simulink model "ManualModel_With_OptiTrack"  (R2025a)
settings: Solver=ode4  StartTime=0  StopTime=inf  FixedStep=0.01  RelTol=1e-3
undefined symbols (not defined in the file): Angular, getRigidBodyPose, Linear, scenario
libraries: robotlib x4, simulink_extras x2, vrlib x1
settings Model: SimulationMode=external  Creator=20212285  LastModifiedBy=jakub
settings SolverCC: AlgebraicLoopSolver=LineSearch
settings DataIOCC: ReturnWorkspaceOutputsName=s
settings OptimizationCC: EnhancedBackFolding=on  PassReuseOutputArgsAs=Individual arguments  ZeroExternalMemoryAtStartup=off  ZeroInternalMemoryAtStartup=off  MaxStackSize=64  OptimizeBlockOrder=speed  DifferentSizesBufferReuse=on  OptimizationCustomize=off  EfficientTunableParamExpr=on
settings DebuggingCC: ParameterTunabilityLossMsg=error  UnconnectedInputMsg=warning  UnconnectedOutputMsg=warning  UnconnectedLineMsg=warning
settings HardwareCC: ProdBitPerPointer=32.0  ProdBitPerSizeT=32.0  ProdBitPerPtrDiffT=32.0  ProdLargestAtomicFloat=None  ProdIntDivRoundTo=Undefined  ProdEndianess=Unspecified  ProdWordSize=32.0  ProdHWDeviceType=Generic->Unspecified (assume 32-bit Generic)
settings ModelReferenceCC: EnableRefExpFcnMdlSchedulingChecks=on
settings SFSimCC: MATLABDynamicMemAlloc=off  SimTargetLang=C++  SimDLTargetLibrary=mkl-dnn
settings RTWCC: SystemTargetFile=ert.tlc  HardwareBoard=Robot Operating System (ROS)  TLCOptions="-aInlineSetEventsForThisBaseRateFcn=TLC_FALSE -aSuppressMultiTaskScheduler=TLC_FALSE  -aRateBasedStepFcn=0"  TemplateMakefile=ert_default_tmf  Toolchain=Catkin  TargetLang=C++  GPUComputeCapability=3.5  Description=Embedded Coder
settings CodeAppCC: ForceParamTrailComments=on  IgnoreCustomStorageClasses=off  OperatorAnnotations=on  SimulinkDataObjDesc=on  SFDataObjDesc=on  InsertBlockDesc=on
settings ERTTargetCC: ExtModeTransport=0.0  ExtModeStaticAlloc=off  ExtModeMexFile=ext_comm  ExtModeIntrfLevel=Level1  InlinedParameterPlacement=Hierarchical  DynamicArrayContainerType=coder::array

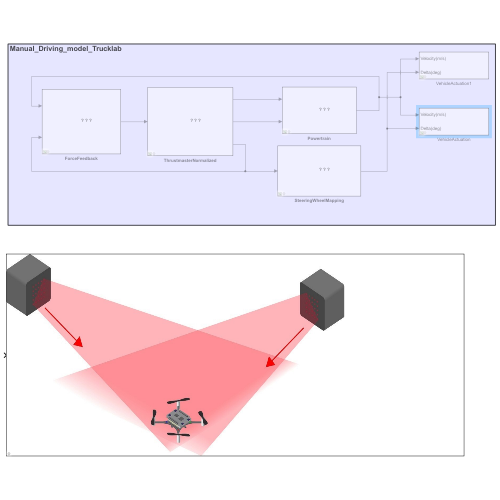
[thumbnail: Simulink's stored preview of the top-level diagram]
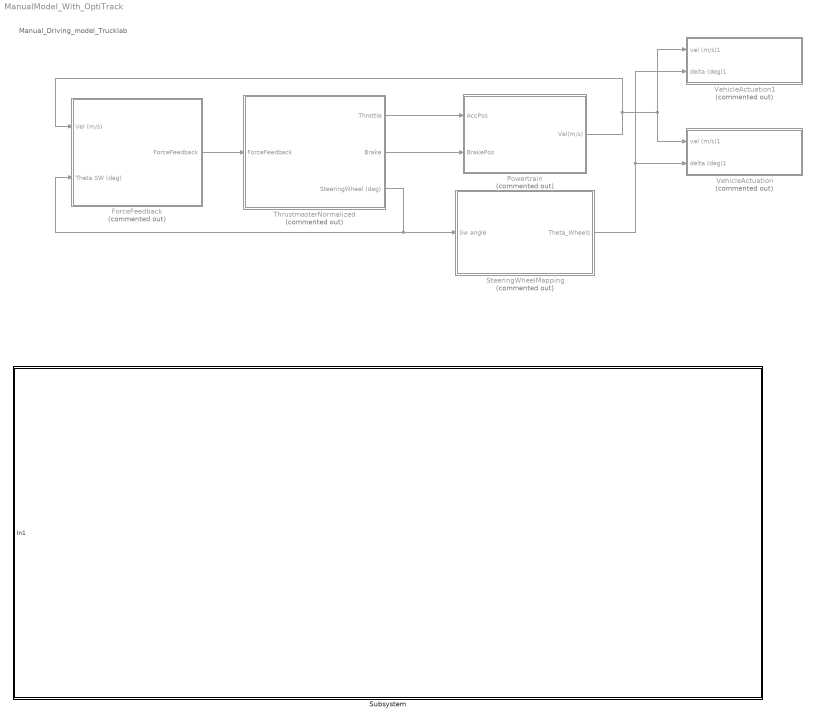
== system ManualModel_With_OptiTrack ==
  note: Manual_Driving_model_Trucklab
  ForceFeedback : Subsystem  Commented=on  mask(Thrustmaster ForceFeedback){}
      mask help:
      | Use this block to give drivers a realistic, centered steer feel: no force at zero.
      |
      | The ForceFeedback block computes a normalized return-to-center torque for a steering wheel. A zero output produces no force; negative values apply maximum rightward torque (–1), and positive values apply maximum leftward torque (+1). Internally, it:
      |
      | Ignores small angles around center (dead-zone)
      | Adds a speed-scaled spring torque pulling the wheel back toward center
      mask Display:
      | image('ForceFeedback.jpg');
      | port_label('input', 1, 'Vel (m/s)')
      | port_label('input', 2, 'Theta_SW (deg)')
      | port_label('output', 1, 'ForceFeedback')
  Powertrain : Subsystem  Commented=on  mask(Powertrain){}
      mask help:
      | Converts driver inputs (Throttle and Brake) and current vehicle speed into longitudinal acceleration. The block outputs a computed acceleration value, which feeds an integrator to produce vehicle velocity, and also outputs a stop_signal that can be used to force the vehicle to halt under very low velocity.
      |
      | Input throttle and brake should be normalized [0,1].
      mask Display:
      | image('Powertrain.jpg');
      | port_label('input', 1, 'Throttle')
      | port_label('input', 2, 'Brake')
      | port_label('output', 1, 'vel (m/s)')
  SteeringWheelMapping : Subsystem  Commented=on  mask(SteeringWheel_Mapping){}
      mask help:
      | SteeringWheel_Mapping maps the raw steering wheel angle (theta_sw) to a modified output (theta_mapped) using one of two modes:
      |
      | Mode = 0 applies a fixed linear gain of 38
      | Mode = 1 applies a nonlinear mapping via the VariableMap function.
      |
      | To change the modes, click the arrow in the bottemleft to open the system, and double-click the manual switch.
      mask Display:
      | image('Steering_mapping.jpg');
      | port_label('input', 1, 'SW_angle (deg)')
      | port_label('output', 1, 'Theta_Wheels (deg)')
  Subsystem : Subsystem
      mask Display: image('optitrack.jpg');
  ThrustmasterNormalized : Subsystem  Commented=on  mask(Thrustmaster_Normalized_Input){}
      mask help:
      | The Thrustmaster_Normalized block converts raw joystick signals from a Thrustmaster wheel‐pedal set into three normalized outputs and one normalized input for force feedback.
      |
      | SteeringWheel output ranges from –450 (full right) to +450 (full left), using standard ISO coordinates (counterclockwise rotation is positive).
      |
      | Pedal (Throttle) output ranges from 0 (no throttle) to 1 (full throttle) using the rightmost pedal.
      |
      | Brake output ranges from 0 (no braking) to 1 (full braking) using the middle pedal.
      |
      | ForceFeedback input accepts a command in the range –1 to +1 to drive the wheel motor.
      mask Display:
      | %image('C:\Users\tarun\OneDrive\Desktop\Flags\thrust.jpg'); % Use "Edit Image" on toolstrip to change.
      | image('joystick.jpg');
      | port_label('input', 1, 'ForceFeedback([-1,1])')
      | port_label('output', 1, 'Throttle[0,1]')
      | port_label('output', 2, 'Brake[0,1]')
      | port_label('output', 3, 'SteeringWheel[-450,450]')
  VehicleActuation : Subsystem  Commented=on  mask(Vehicle Actuation){robotIndex=1, topic=/tractor1/cmd, messageType=geometry_msgs/Twist}
      mask prompts: robotIndex "Type the Index no."; topic "ros:slros:blockmask:TopicPrompt"; messageType "ros:slros:blockmask:MessageTypePrompt"
      mask help:
      | The velocity and steering angle inputs from the Thrustmaster Input block are published to a ROS topic. A ROS node on the actuator hardware side subscribes to this topic and executes the corresponding control actions.
      |
      | Select the tractor index that you wish to control.
      mask init:
      | % Retrieve mask parameters
      | robotIndex = str2double(get_param(gcb, 'robotIndex')); % Get the robot index
      |          % Get the topic source, if applicable
      | 
      | % Define the base path for the ROS blocks inside the subsystem
      | 
      | publishBlockPath = strcat(gcb);       % Adjust path for ROS Publish block
      | 
      | 
      | 
      | % For ROS Publish block
      | pubTopic = sprintf('/tractor%d/cmd', robotIndex);     % Example topic for Publish
      | set_param(publishBlockPath, 'Topic', pubTopic);
      | set_param(publishBlockPath, 'MessageType', 'geometry_msgs/Twist');
      mask Help:
      | Description:
      | <p style="font-family: Arial, sans-serif; font-size: 12px;"> The <b>Vehicle Actuation Block</b> provides an interface to control the physical actuators of the trucks in the <b>TruckLab</b> environment. It accepts <b>velocity (in m/s)</b> and <b>steering angle (in radians)</b> as inputs and publishes these control signals to the ROS network via the <b>ROS Publish Block</b>. </p>
      | Inputs:
      | <ul style="font-family: Arial, sans-serif; font-size: 12px;"> <li><b>Velocity (m/s):</b> Desired velocity of the truck.</li> <li><b>Steering Angle (rad):</b> Desired steering angle of the truck.</li> </ul>
      | Outputs:
      | <ul style="font-family: Arial, sans-serif; font-size: 12px;"> <li><b>ROS Message:</b> The block publishes a <b>geometry_msgs/Twist</b> message to the ROS topic <code>/tractor&lt;ID&gt;/cmd</code>, where <code>&lt;ID&gt;</code> is the truck number. The message contains: <ul> <li><b>Linear.X:</b> Velocity (m/s).</li> <li><b>Angular.Z:</b> Steering angle (rad).</li> </ul> </li> </ul>
      | Parameters:
      | <ul style="font-family: Arial, sans-serif; font-size: 12px;"> <li><b>Truck Number:</b> The ID of the truck to be controlled (e.g., 1, 2, 3). This dynamically updates the ROS topic name (e.g., <code>/tractor3/cmd</code>).</li> </ul>
      | Functionality:
      | <ol style="font-family: Arial, sans-serif; font-size: 12px;"> <li><b>Input Signals:</b> <ul> <li>The block accepts two input signals: <ul> <li><b>Velocity (m/s):</b> Controls the truck's speed.</li> <li><b>Steering Angle (rad):</b> Controls the truck's direction.</li> </ul> </li> </ul> </li> <li><b>ROS Message Setup:</b> <ul> <li>A <b>ROS Blank Message Block</b> generates a blank <b>geometry_msgs/Twist</b> message. This message type is standard for controlling mobile robots and contains two main fields: <ul> <li><b>Linear:</b> For translational motion (velocity).</li> <li><b>Angular:</b> For rotational motion (steering).</li> </ul> </li> </ul> </li> <li><b>Populating the Message:</b> <ul> <li>A <b>Bus Assignment Block</b> is used to assign the input signals to the appropriate fields in the <b>geometry_msgs/Twist</b> message: <ul> <li><b>Linear.X:</b> Assigned to the velocity input.</li> <li><b>Angular.Z:</b> Assigned to the steering angle input.</li> </ul> </li> </ul> </li> <li><b>Publishing to ROS:</b> <ul> <li>The populated message is published to the ROS topic <code>/tractor&lt;ID&gt;/cmd</code> using the <b>ROS Publish Block</b>, where <code>&lt;ID&gt;</code> is the truck number. This allows real-time control of the truck's movement.</li> </ul> </li> <li><b>Dynamic Topic Naming:</b> <ul> <li>The ROS topic name is dynamically updated based on the selected truck number (e.g., <code>/tractor3/cmd</code> for truck 3).</li> </ul> </li> </ol>
      | User Instructions:
      | <ol style="font-family: Arial, sans-serif; font-size: 12px;"> <li>Add the <b>Vehicle Actuation Block</b> to your Simulink model.</li> <li>Set the <b>Truck Number</b> parameter to match the ID of the truck you want to control.</li> <li>Connect the <b>velocity (m/s)</b> and <b>steering angle (rad)</b> signals to the block inputs.</li> <li>Run the model to publish control signals to the ROS network.</li> </ol>
      | Example Usage:
      | <p style="font-family: Arial, sans-serif; font-size: 12px;"> To control <b>Tractor 3</b>, set the <b>Truck Number</b> to 3. The block will publish velocity and steering angle commands to the ROS topic <code>/tractor3/cmd</code>. </p>
      | References:
      | <ul style="font-family: Arial, sans-serif; font-size: 12px;"> <li><b>ROS Publish Block Documentation:</b> <a href="https://nl.mathworks.com/help/ros/ref/publish.html">https://nl.mathworks.com/help/ros/ref/publish.html</a></li> <li><b>ROS Blank Message Block Documentation:</b> <a href="https://nl.mathworks.com/help/ros/ref/blankmessage.html">https://nl.mathworks.com/help/ros/ref/blankmessage.html</a></li> </ul>
      mask TypeOptions topic: Publish1/topic
      mask TypeOptions messageType: Publish1/messageType
      mask DialogControl topic Prompt: Topic:
      mask DialogControl messageType Prompt: Message type:
      mask Display:
      | port_label('input', 1, 'Velocity(m/s)')
      | port_label('input', 2, 'Delta(deg)')
  VehicleActuation1 : Subsystem  Commented=on  mask(Vehicle Actuation){robotIndex=1, topic=/tractor1/cmd, messageType=geometry_msgs/Twist}
      mask prompts: robotIndex "Type the Index no."; topic "ros:slros:blockmask:TopicPrompt"; messageType "ros:slros:blockmask:MessageTypePrompt"
      mask help:
      | The velocity and steering angle inputs from the Thrustmaster Input block are published to a ROS topic. A ROS node on the actuator hardware side subscribes to this topic and executes the corresponding control actions.
      |
      | Select the tractor index that you wish to control.
      mask init:
      | % Retrieve mask parameters
      | robotIndex = str2double(get_param(gcb, 'robotIndex')); % Get the robot index
      |          % Get the topic source, if applicable
      | 
      | % Define the base path for the ROS blocks inside the subsystem
      | 
      | publishBlockPath = strcat(gcb);       % Adjust path for ROS Publish block
      | 
      | 
      | 
      | % For ROS Publish block
      | pubTopic = sprintf('/tractor%d/cmd', robotIndex);     % Example topic for Publish
      | set_param(publishBlockPath, 'Topic', pubTopic);
      | set_param(publishBlockPath, 'MessageType', 'geometry_msgs/Twist');
      mask Help:
      | Description:
      | <p style="font-family: Arial, sans-serif; font-size: 12px;"> The <b>Vehicle Actuation Block</b> provides an interface to control the physical actuators of the trucks in the <b>TruckLab</b> environment. It accepts <b>velocity (in m/s)</b> and <b>steering angle (in radians)</b> as inputs and publishes these control signals to the ROS network via the <b>ROS Publish Block</b>. </p>
      | Inputs:
      | <ul style="font-family: Arial, sans-serif; font-size: 12px;"> <li><b>Velocity (m/s):</b> Desired velocity of the truck.</li> <li><b>Steering Angle (rad):</b> Desired steering angle of the truck.</li> </ul>
      | Outputs:
      | <ul style="font-family: Arial, sans-serif; font-size: 12px;"> <li><b>ROS Message:</b> The block publishes a <b>geometry_msgs/Twist</b> message to the ROS topic <code>/tractor&lt;ID&gt;/cmd</code>, where <code>&lt;ID&gt;</code> is the truck number. The message contains: <ul> <li><b>Linear.X:</b> Velocity (m/s).</li> <li><b>Angular.Z:</b> Steering angle (rad).</li> </ul> </li> </ul>
      | Parameters:
      | <ul style="font-family: Arial, sans-serif; font-size: 12px;"> <li><b>Truck Number:</b> The ID of the truck to be controlled (e.g., 1, 2, 3). This dynamically updates the ROS topic name (e.g., <code>/tractor3/cmd</code>).</li> </ul>
      | Functionality:
      | <ol style="font-family: Arial, sans-serif; font-size: 12px;"> <li><b>Input Signals:</b> <ul> <li>The block accepts two input signals: <ul> <li><b>Velocity (m/s):</b> Controls the truck's speed.</li> <li><b>Steering Angle (rad):</b> Controls the truck's direction.</li> </ul> </li> </ul> </li> <li><b>ROS Message Setup:</b> <ul> <li>A <b>ROS Blank Message Block</b> generates a blank <b>geometry_msgs/Twist</b> message. This message type is standard for controlling mobile robots and contains two main fields: <ul> <li><b>Linear:</b> For translational motion (velocity).</li> <li><b>Angular:</b> For rotational motion (steering).</li> </ul> </li> </ul> </li> <li><b>Populating the Message:</b> <ul> <li>A <b>Bus Assignment Block</b> is used to assign the input signals to the appropriate fields in the <b>geometry_msgs/Twist</b> message: <ul> <li><b>Linear.X:</b> Assigned to the velocity input.</li> <li><b>Angular.Z:</b> Assigned to the steering angle input.</li> </ul> </li> </ul> </li> <li><b>Publishing to ROS:</b> <ul> <li>The populated message is published to the ROS topic <code>/tractor&lt;ID&gt;/cmd</code> using the <b>ROS Publish Block</b>, where <code>&lt;ID&gt;</code> is the truck number. This allows real-time control of the truck's movement.</li> </ul> </li> <li><b>Dynamic Topic Naming:</b> <ul> <li>The ROS topic name is dynamically updated based on the selected truck number (e.g., <code>/tractor3/cmd</code> for truck 3).</li> </ul> </li> </ol>
      | User Instructions:
      | <ol style="font-family: Arial, sans-serif; font-size: 12px;"> <li>Add the <b>Vehicle Actuation Block</b> to your Simulink model.</li> <li>Set the <b>Truck Number</b> parameter to match the ID of the truck you want to control.</li> <li>Connect the <b>velocity (m/s)</b> and <b>steering angle (rad)</b> signals to the block inputs.</li> <li>Run the model to publish control signals to the ROS network.</li> </ol>
      | Example Usage:
      | <p style="font-family: Arial, sans-serif; font-size: 12px;"> To control <b>Tractor 3</b>, set the <b>Truck Number</b> to 3. The block will publish velocity and steering angle commands to the ROS topic <code>/tractor3/cmd</code>. </p>
      | References:
      | <ul style="font-family: Arial, sans-serif; font-size: 12px;"> <li><b>ROS Publish Block Documentation:</b> <a href="https://nl.mathworks.com/help/ros/ref/publish.html">https://nl.mathworks.com/help/ros/ref/publish.html</a></li> <li><b>ROS Blank Message Block Documentation:</b> <a href="https://nl.mathworks.com/help/ros/ref/blankmessage.html">https://nl.mathworks.com/help/ros/ref/blankmessage.html</a></li> </ul>
      mask TypeOptions topic: Publish1/topic
      mask TypeOptions messageType: Publish1/messageType
      mask DialogControl topic Prompt: Topic:
      mask DialogControl messageType Prompt: Message type:
      mask Display:
      | port_label('input', 1, 'Velocity(m/s)')
      | port_label('input', 2, 'Delta(deg)')
  wires:
  ThrustmasterNormalized/1(Throttle) -> Powertrain/1(AccPos)
  ThrustmasterNormalized/2(Brake) -> Powertrain/2(BrakePos)
  ThrustmasterNormalized/3(SteeringWheel (deg)) -> ForceFeedback/2(Theta SW (deg)), SteeringWheelMapping/1(Sw angle)
  ForceFeedback/1(ForceFeedback) -> ThrustmasterNormalized/1(ForceFeedback)
  Powertrain/1(Vel(m/s)) -> ForceFeedback/1(Vel (m/s)), VehicleActuation/1(vel (m/s)1), VehicleActuation1/1(vel (m/s)1)
  SteeringWheelMapping/1(Theta_Wheels) -> VehicleActuation/2(delta (deg)1), VehicleActuation1/2(delta (deg)1)

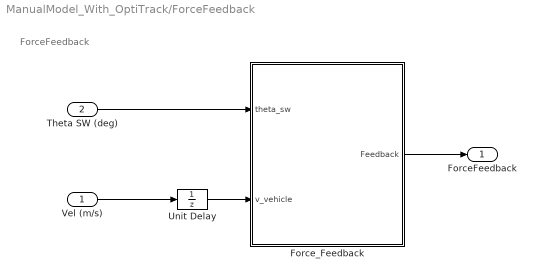
== system ManualModel_With_OptiTrack/ForceFeedback ==
  note: ForceFeedback
  Vel (m/s) : Inport
  Theta SW (deg) : Inport  Port=2
  Force_Feedback : MATLAB Function  TreatAsAtomicUnit=on
  Unit Delay : UnitDelay  SampleTime=-1  HasFrameUpgradeWarning=on
  ForceFeedback : Outport
  wires:
  Theta SW (deg)/1 -> Force_Feedback/1(theta_sw)
  Force_Feedback/1(Feedback) -> ForceFeedback/1
  Vel (m/s)/1 -> Unit Delay/1
  Unit Delay/1 -> Force_Feedback/2(v_vehicle)

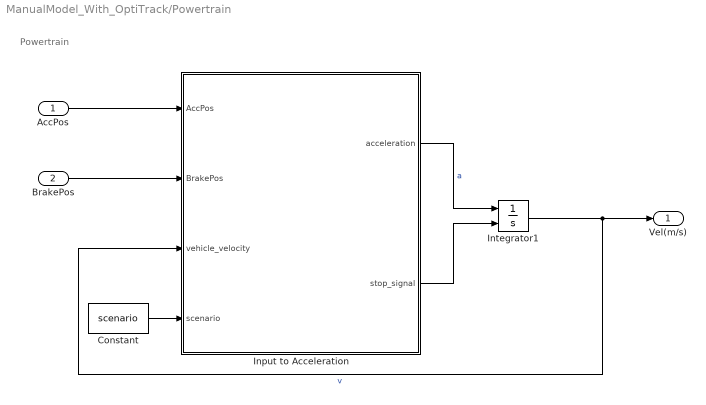
== system ManualModel_With_OptiTrack/Powertrain ==
  note: Powertrain
  AccPos : Inport
  BrakePos : Inport  Port=2
  Constant : Constant  InitFcn=|  Value=scenario
      | % ==== Scenario chooser dialog ====
      | choice = questdlg( ...
      |   'Select vehicle scenario:', ...
      |   'Vehicle Configuration', ...
      |   '1) Tractor only','2) Tractor + empty trailer','3) Tractor + loaded trailer', ...
      |   '1) Tractor only' );
      | 
      | % Map the user’s choice to an integer
      | switch choice
      |   case '1) Tractor only'
      |     scenario = 1;
      |   case '2) Tractor + empty trailer'
      |     scenario = 2;
      |   case '3) Tractor + loaded trailer'
      |     scenario = 3;
      |   otherwise
      |     scenario = 1;
      | end
      | 
      | % Push into base workspace
      | assignin('base','scenario',scenario);
  Input to Acceleration : MATLAB Function  TreatAsAtomicUnit=on
  Integrator1 : Integrator  ExternalReset=level
  Vel(m/s) : Outport
  wires:
  BrakePos/1 -> Input to Acceleration/2(BrakePos)
  Constant/1 -> Input to Acceleration/4(scenario)
  AccPos/1 -> Input to Acceleration/1(AccPos)
  Input to Acceleration/2(stop_signal) -> Integrator1/2
  Input to Acceleration/1(acceleration) -> Integrator1/1  "a"
  Integrator1/1 -> Input to Acceleration/3(vehicle_velocity), Vel(m/s)/1  "v"

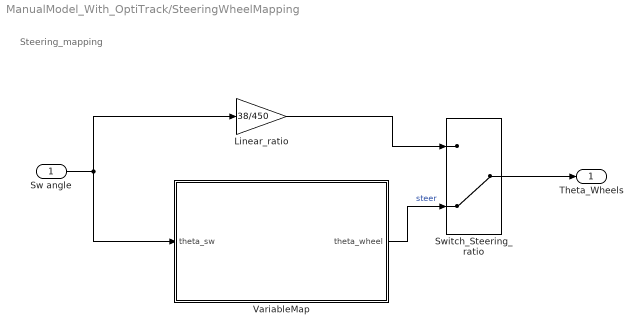
== system ManualModel_With_OptiTrack/SteeringWheelMapping ==
  note: Steering_mapping
  Sw angle : Inport
  Linear_ratio : Gain  Gain=38/450
  Switch_Steering_ratio : ManualSwitch  CurrentSetting=0
  VariableMap : MATLAB Function  TreatAsAtomicUnit=on
  Theta_Wheels : Outport
  wires:
  Sw angle/1 -> Linear_ratio/1, VariableMap/1("theta_sw ")
  Linear_ratio/1 -> Switch_Steering_ratio/1
  Switch_Steering_ratio/1 -> Theta_Wheels/1
  VariableMap/1(theta_wheel) -> Switch_Steering_ratio/2  "steer"

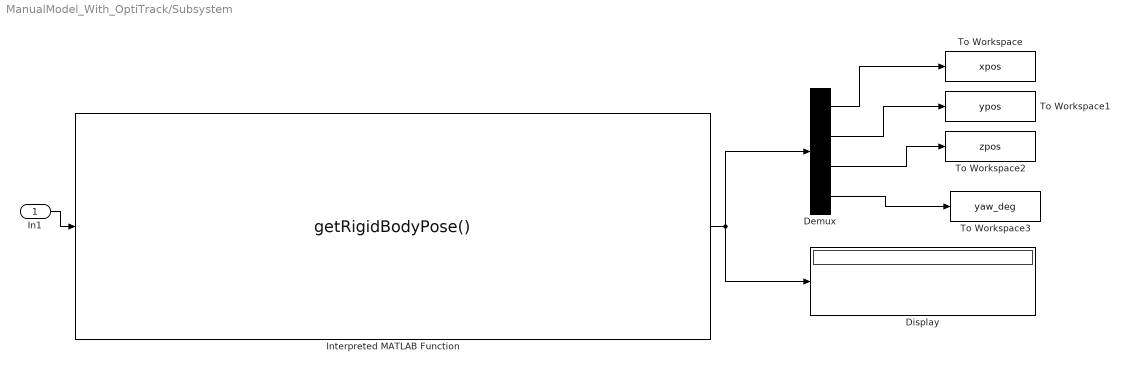
== system ManualModel_With_OptiTrack/Subsystem ==
  In1 : Inport
  Demux : Demux
  Display : Display
  Interpreted MATLAB Function : MATLABFcn  MATLABFcn=getRigidBodyPose()
  To Workspace : ToWorkspace  VariableName=xpos  SaveFormat=Timeseries  SampleTime=-1
  To Workspace1 : ToWorkspace  VariableName=ypos  SaveFormat=Timeseries  SampleTime=-1
  To Workspace2 : ToWorkspace  VariableName=zpos  SaveFormat=Timeseries  SampleTime=-1
  To Workspace3 : ToWorkspace  VariableName=yaw_deg  SaveFormat=Timeseries  SampleTime=-1
  wires:
  Interpreted MATLAB Function/1 -> Demux/1, Display/1
  Demux/2 -> To Workspace1/1
  Demux/4 -> To Workspace3/1
  Demux/1 -> To Workspace/1
  In1/1 -> Interpreted MATLAB Function/1
  Demux/3 -> To Workspace2/1

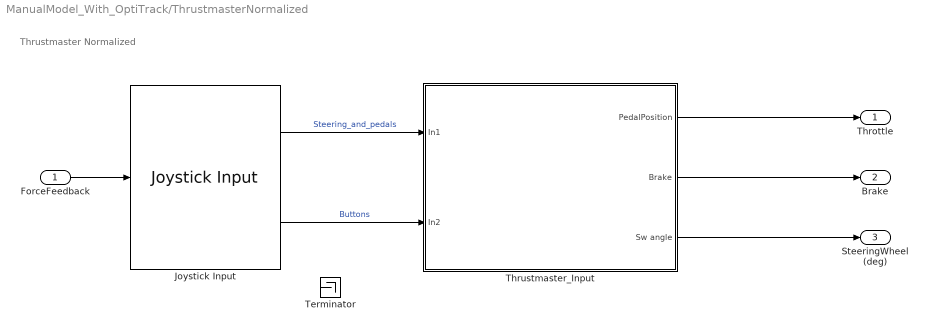
== system ManualModel_With_OptiTrack/ThrustmasterNormalized ==
  note: Thrustmaster Normalized
  ForceFeedback : Inport
  Joystick Input : vrlib/Joystick Input  joyid=1  adjustports=on  forcefeed=on  mask(Joystick Input){}
      mask Display: image('joystick.jpg'); % Use "Edit Image" on toolstrip to change.
  Terminator : Terminator
  Thrustmaster_Input : Subsystem
  Throttle : Outport
  Brake : Outport  Port=2
  SteeringWheel (deg) : Outport  Port=3
  wires:
  ? -> Terminator/1
  ForceFeedback/1 -> Joystick Input/1
  Thrustmaster_Input/3(Sw angle) -> SteeringWheel (deg)/1
  Thrustmaster_Input/2(Brake) -> Brake/1
  Joystick Input/1 -> Thrustmaster_Input/1(In1)  "Steering_and_pedals"
  Joystick Input/2 -> Thrustmaster_Input/2(In2)  "Buttons"
  Thrustmaster_Input/1(PedalPosition) -> Throttle/1

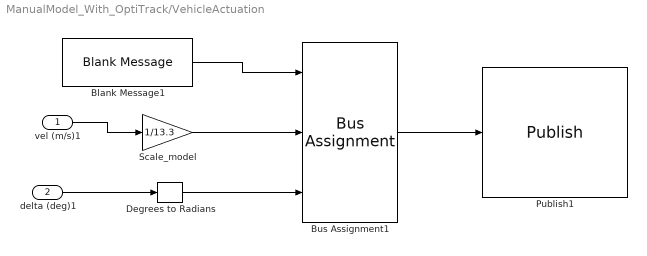
== system ManualModel_With_OptiTrack/VehicleActuation ==
  vel (m/s)1 : Inport
  delta (deg)1 : Inport  Port=2
  Blank Message1 : robotlib/Blank Message  messageClass=Message  entityType=geometry_msgs/Twist  messageType=geometry_msgs/Twist  SampleTime=-1  legacyBusStruct=off
  Bus Assignment1 : BusAssignment  DialogController=Simulink.DDGSource_BusAssignment  AssignedSignals=Linear.X,Angular.Z
  Degrees to Radians : simulink_extras/Transformations/Degrees to Radians
  Publish1 : robotlib/Publish  topicSource=Select from ROS network  topic=/tractor1/cmd  messageType=geometry_msgs/Twist  legacyBusStruct=off  messageQueueLength=1
      link override SinkBlock: ROSTopic=/cmd_vel  ROSMessageType=geometry_msgs/Twist  SLBusName=SL_Bus_TruckLab_MannualDrivingROS1_geometry_msgs_Twist  ModelName=TruckLab_MannualDrivingROS1  BlockId=Pub_TruckLab_MannualDrivingROS1_402
  Scale_model : Gain  Gain=1/13.3
  wires:
  Blank Message1/1 -> Bus Assignment1/1
  Degrees to Radians/1 -> Bus Assignment1/3
  Scale_model/1 -> Bus Assignment1/2
  Bus Assignment1/1 -> Publish1/1
  delta (deg)1/1 -> Degrees to Radians/1
  vel (m/s)1/1 -> Scale_model/1

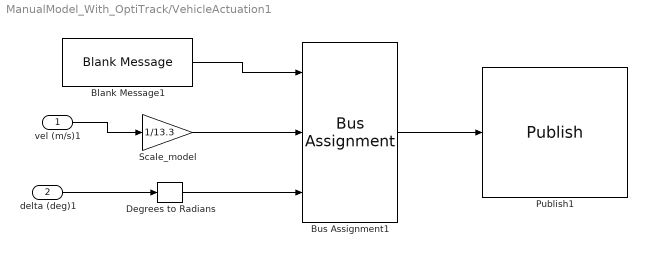
== system ManualModel_With_OptiTrack/VehicleActuation1 ==
  vel (m/s)1 : Inport
  delta (deg)1 : Inport  Port=2
  Blank Message1 : robotlib/Blank Message  messageClass=Message  entityType=geometry_msgs/Twist  messageType=geometry_msgs/Twist  SampleTime=-1  legacyBusStruct=off
  Bus Assignment1 : BusAssignment  DialogController=Simulink.DDGSource_BusAssignment  AssignedSignals=Linear.X,Angular.Z
  Degrees to Radians : simulink_extras/Transformations/Degrees to Radians
  Publish1 : robotlib/Publish  topicSource=Specify your own  topic=/tractor1/cmd  messageType=geometry_msgs/Twist  legacyBusStruct=off  messageQueueLength=1
      link override SinkBlock: ROSTopic=/cmd_vel  ROSMessageType=geometry_msgs/Twist  SLBusName=SL_Bus_TruckLab_MannualDrivingROS1_geometry_msgs_Twist  ModelName=TruckLab_MannualDrivingROS1  BlockId=Pub_TruckLab_MannualDrivingROS1_402
  Scale_model : Gain  Gain=1/13.3
  wires:
  vel (m/s)1/1 -> Scale_model/1
  delta (deg)1/1 -> Degrees to Radians/1
  Bus Assignment1/1 -> Publish1/1
  Scale_model/1 -> Bus Assignment1/2
  Degrees to Radians/1 -> Bus Assignment1/3
  Blank Message1/1 -> Bus Assignment1/1

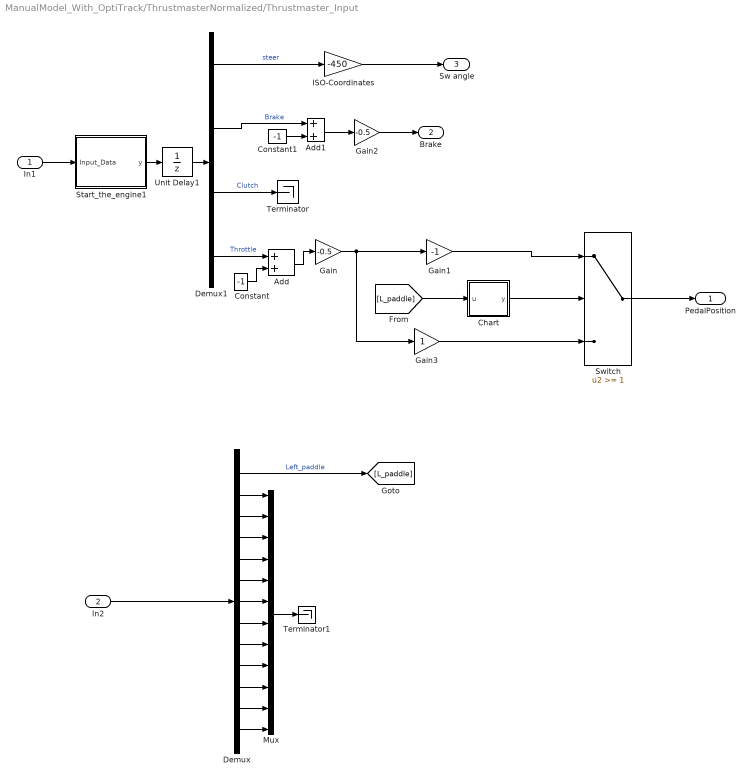
== system ManualModel_With_OptiTrack/ThrustmasterNormalized/Thrustmaster_Input ==
  In1 : Inport
  In2 : Inport  Port=2
  Add : Sum
  Add1 : Sum
  Chart : Stateflow chart  TreatAsAtomicUnit=on
  Constant : Constant  Value=-1
  Constant1 : Constant  Value=-1
  Demux : Demux  Outputs=13
  Demux1 : Demux
  Gain : Gain  Gain=-0.5
  Gain1 : Gain  Gain=-1
  Gain2 : Gain  Gain=-0.5
  Gain3 : Gain
  ISO-Coordinates : Gain  Gain=-450
  Mux : Mux  Inputs=12
  Start_the_engine1 : Stateflow chart  TreatAsAtomicUnit=on
  Switch : Switch  Threshold=1  SaturateOnIntegerOverflow=off  InputSameDT=off
  Terminator : Terminator
  Terminator1 : Terminator
  Unit Delay1 : UnitDelay  SampleTime=-1  HasFrameUpgradeWarning=on
  PedalPosition : Outport
  Brake : Outport  Port=2
  Sw angle : Outport  Port=3
  wires:
  Unit Delay1/1 -> Demux1/1
  Start_the_engine1/1(y) -> Unit Delay1/1
  [L_paddle] -> Chart/1(u)
  Demux/7 -> Mux/6
  Demux1/1 -> ISO-Coordinates/1  "steer"
  Demux/3 -> Mux/2
  Demux/4 -> Mux/3
  Demux/2 -> Mux/1
  Mux/1 -> Terminator1/1
  Switch/1 -> PedalPosition/1
  In1/1 -> Start_the_engine1/1(Input_Data)
  Demux/13 -> Mux/12
  Demux/1 -> [L_paddle]  "Left_paddle"
  Demux/5 -> Mux/4
  Demux/11 -> Mux/10
  In2/1 -> Demux/1
  Demux1/2 -> Add1/1  "Brake"
  Demux/12 -> Mux/11
  Demux/8 -> Mux/7
  Demux/10 -> Mux/9
  Add1/1 -> Gain2/1
  ISO-Coordinates/1 -> Sw angle/1
  Demux/6 -> Mux/5
  Gain3/1 -> Switch/3
  Gain2/1 -> Brake/1
  Gain1/1 -> Switch/1
  Demux/9 -> Mux/8
  Demux1/3 -> Terminator/1  "Clutch"
  Constant1/1 -> Add1/2
  Demux1/4 -> Add/1  "Throttle"
  Chart/1(y) -> Switch/2
  Constant/1 -> Add/2
  Add/1 -> Gain/1
  Gain/1 -> Gain1/1, Gain3/1

== stateflow chart ManualModel_With_OptiTrack/ThrustmasterNormalized/Thrustmaster_Input/Chart ==
  state Wait1
    y=0;
  state Neutral
    y=0;
  state Wait_for_start
    y=0;
  state Forward
    entry: y=1;
  state Reverse
    entry: y=-1;
  state Wait
    y=0;
  (default) -> Neutral
  Wait1 -> Reverse : [u<0.5]
  Forward -> Wait1 : [u>0.5]
  Neutral -> Wait_for_start : [u>0.5]
  Wait_for_start -> Forward : [u<0.5]
  Wait -> Forward : [u<0.5]
  Reverse -> Wait : [u>0.5]
  data: u input; y output

== matlab function ManualModel_With_OptiTrack/Powertrain/Input to Acceleration ==
  data: acceleration output; stop_signal output; AccPos input; BrakePos input; vehicle_velocity input; scenario input
function [acceleration, stop_signal] = Input_to_acceleration(AccPos, BrakePos, vehicle_velocity, scenario)
% Scenarios: total mass & drive-axle load
switch scenario
    case 1  % tractor only
        total_mass     = 8000;         % [kg] 
        drive_load_mass= 2400;         % [kg] on rear axle
        C_rr           = 0.006;
    case 2  % tractor + empty trailer
        total_mass     = 15200;        % [kg]
        drive_load_mass= 3600;         % [kg] on rear axle
        C_rr           = 0.006;        
    case 3  % tractor + heavy trailer
        total_mass     = 40000;        % [kg] 
        drive_load_mass= 10600;        % [kg] weight on axle
        C_rr           = 0.006;
    otherwise
        error('scenario must be 1,2 or 3')
end    

% Vehicle Parameters
T_max        = 2300;        % Max motor torque [Nm]
T_ramp_start = 1000;        % Torque at start[Nm]
eff          = 0.90;        % Efficiency
g            = 9.81;        % Gravity [m/s^2]
vel_thresh   = 0.0001;       % stop
% Drivetrain
tire_radius = 0.552;       % Wheel radius [m]
ratio       = 8;           % Gear ratio
 
% Ramp & decay settings
RPM_ramp            = 200;  % End of ramp region [RPM]
RPM_break_simulated = 538;  % Start of linear decay [RPM]
decay_slope         = 17.5; % Nm drop per RPM beyond break
v_limit             = 15/3.6;% Top speed [m/s]
engine_brake_p      = 0.3;  % Factor peak engine brake- of motor peak Torque
% Convert vehicle speed to engine RPM
RPM         = (abs(vehicle_velocity) * ratio) / (2*pi*tire_radius) * 60; 
stop_signal = 0;

% Motor torque
if RPM <= RPM_ramp
    T_motor = T_ramp_start + (T_max - T_ramp_start) * (RPM / RPM_ramp);
elseif RPM <= RPM_break_simulated
    T_motor = T_max;
elseif vehicle_velocity <= v_limit
    T_motor = T_max - decay_slope * (RPM - RPM_break_simulated);
else
    T_motor = 0;           % coast above 15km/h
end

% Traction limit based on rear-axle load
mu         = 0.8;                           % friction coefficient
F_grip_max = mu * drive_load_mass * g;      % traction limit
T_grip_max = (F_grip_max * tire_radius) / ratio;

% Apply pedal position and efficiency
T_req           = T_motor * AccPos * eff;
T_motor_actual  = sign(T_req) * min(abs(T_req), T_grip_max);

% Resistive forces
F_trac = (T_motor_actual * ratio) / tire_radius;
if abs(vehicle_velocity) > vel_thresh
    F_roll = -sign(vehicle_velocity) * total_mass * g * C_rr;
else
    F_roll = 0;
    if AccPos == 0
        stop_signal = 1;
    end
end

% Engine braking
target_velocity = AccPos * v_limit;
if (abs(vehicle_velocity) > abs(target_velocity)) && (AccPos < 1) % only when pedal is not flat out.
    if abs(vehicle_velocity) <= 1 
        T_eb_max = (T_max/1) * abs(vehicle_velocity);
    else
        T_eb_max = abs(T_max); 
    end
else
    T_eb_max = 0;
end  

T_eb_max = engine_brake_p* T_eb_max;
F_eb = -sign(vehicle_velocity) * ( T_eb_max * ratio / tire_radius) * (1 - AccPos); 


%Braking using an target deceleration
a_brake_max = 6;                        %m/s
if BrakePos> 0
    a_target    = BrakePos * a_brake_max;                               %mapping of pedal
    F_brake_req = (total_mass * a_target) - abs(F_roll) - abs(F_eb);    %compute the force needed
    F_brake     = -sign(vehicle_velocity) * F_brake_req;
else
    F_brake =0;
end

% Net force and acceleration (with top‑speed limit)
if (AccPos == 1) && (abs(vehicle_velocity) >= v_limit) && (BrakePos ==0)
    F_net = 0;
elseif (abs(vehicle_velocity) < vel_thresh) && (AccPos ==0)
    F_net = 0;
    stop_signal = 1;
else
    F_net = F_trac + F_roll + F_eb + F_brake;
end
acceleration = F_net / total_mass;

end

== matlab function ManualModel_With_OptiTrack/ForceFeedback/Force_Feedback ==
  data: theta_sw input; v_vehicle input; Feedback output
function Feedback = fcn(theta_sw, v_vehicle)
    % variables
    dead_zone    = 10;        % deg: ignore angles around center
    theta_max    = 1;         % deg: full-lock steering span
    v_max        = 15/3.6;    % m/s: top speed (15 km/h)
    min_torque   = 0.25;      % minimum force to move the wheel
    max_torque   = 0.27;      % maximum feedback force

    % zero feedback if we're close to center
    if abs(theta_sw) <= dead_zone
        Feedback = 0;
    else
        
        % spring force pulling back to center, scaled by vehicle speed
        speed_frac = min(abs(v_vehicle)/v_max, 1);
        if speed_frac > 0
            % ramp torque from min to max 
            t_ramp = min_torque + (max_torque - min_torque) * (abs(theta_sw) / theta_max);
            t_ramp = min(t_ramp, max_torque);
            fs = -sign(theta_sw) * speed_frac * t_ramp;
        else
            fs = 0;
        end

        % combine brake
        rawFb = fs;
        Feedback = max(min(rawFb,  max_torque), -max_torque);
    end
end

== matlab function ManualModel_With_OptiTrack/SteeringWheelMapping/VariableMap ==
  data: theta_sw input; theta_wheel output
function theta_wheel   = variable_steering_ratio(theta_sw)
% VARIABLE_STEERING_RATIO, normalized steering input (-1,1) to wheel angle with variable ratio
c1 = 1/20;                        % 20:1 at center
c3 = (38 - c1*450)/(450^3);       

theta_wheel    = c1*theta_sw + c3*theta_sw.^3;

end

== stateflow chart ManualModel_With_OptiTrack/ThrustmasterNormalized/Thrustmaster_Input/Start_the_engine1 ==
  state Wait
    y= [0; 1; 1; 1];
  state idle
    entry:
    y= [0; 1; 1; 1];
  state Started
    during:
    y = Input_Data;
  (default) -> Wait
  Wait -> idle : after(2, sec)
  idle -> Started : [abs(Input_Data(1)) > 1e-3 || abs(Input_Data(2)) > 1e-3 || abs(Input_Data(3)) > 1e-3 || abs(Input_Data(4)) > 1e-3]
  data: Input_Data input double size=[4 1]; y output double size=[4 1]
